simulink model "RLCCircuit"  (R2023b)
settings: Solver=VariableStepAuto  StartTime=0.0  StopTime=inf  MaxStep=1e-5  RelTol=1e-3
libraries: nesl_utility x6, fl_lib x4, ee_lib x3
settings Model: PacingRate=0.001000  Creator=Rocksmithed  LastModifiedBy=callie
settings DebuggingCC: UnconnectedInputMsg=warning  UnconnectedOutputMsg=warning  UnconnectedLineMsg=warning
settings ModelReferenceCC: EnableRefExpFcnMdlSchedulingChecks=on
settings RTWCC: DLArmComputeVersion=19.05

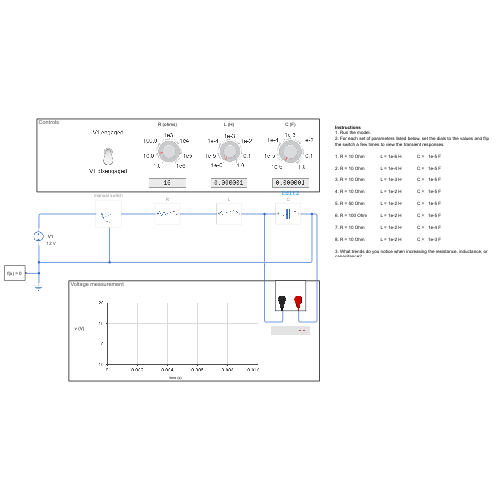
[thumbnail: Simulink's stored preview of the top-level diagram]
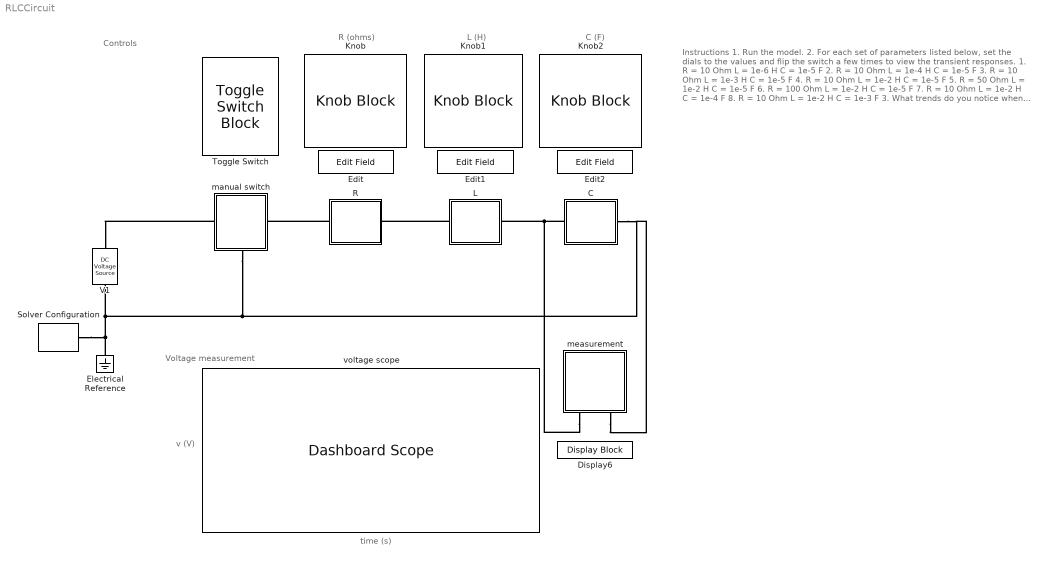
== system RLCCircuit ==
  note: R (ohms)
  note: Voltage measurement
  note: Instructions
      | 1. Run the model.
      | 2. For each set of parameters listed below, set the dials to the values and flip the switch a few times to view the transient responses.
      |
      | 1. R = 10 Ohm L = 1e-6 H C = 1e-5 F
      |
      | 2. R = 10 Ohm L = 1e-4 H C = 1e-5 F
      |
      | 3. R = 10 Ohm L = 1e-3 H C = 1e-5 F
      |
      | 4. R = 10 Ohm L = 1e-2 H C = 1e-5 F
      |
      | 5. R = 50 Ohm L = 1e-2 H C = 1e-5 F
      |
      | 6. R = 100 Ohm L = 1e-2 H C = 1e-5 F
      |
      | 7. R = 10 Ohm L = 1e-2 H C = 1e-4 F
      |
      | 8. R = 10 Ohm L = 1e-2 H C = 1e-3 F
      |
      | 3. What trends do you notice when increasing the resistance, inductance, or capacitance?
  note: time (s)
  note: v (V)
  note: Controls
  note: L (H)
  note: C (F)
  C : Subsystem
      mask Display: image('variablecapacitor.png');
  Display6 : DisplayBlock  LabelPosition=Hide  Format=Custom  Alignment=Right  Transparency=1  FormatString=%0.4f
  Edit : EditField  LabelPosition=Hide  ShowInitialText=on  Alignment=Center
  Edit1 : EditField  LabelPosition=Hide  ShowInitialText=on  Alignment=Center
  Edit2 : EditField  LabelPosition=Hide  ShowInitialText=on  Alignment=Center
  Electrical Reference : fl_lib/Electrical/Electrical Elements/Electrical Reference
  Knob : KnobBlock  LabelPosition=Hide  ScaleMin=1  ScaleMax=1e6  ScaleType=Log
  Knob1 : KnobBlock  LabelPosition=Hide  ScaleMin=1e-6  ScaleMax=1  ScaleType=Log
  Knob2 : KnobBlock  LabelPosition=Hide  ScaleMin=1e-6  ScaleMax=1  ScaleType=Log
  L : Subsystem
      mask Display: image('variableinductor.png');
  R : Subsystem
      mask Display: image('variableresistor.png');
  Solver Configuration : nesl_utility/Solver Configuration  PhysicalDomain=network_engine_domain  SubClassName=solver  LeftPortType=input  RightPortType=generic  Tones=[]  Harmonics=[]  SimulateNoise=off  Profile=off  UseLocalSampling=off  EnableSwitchedLinearOptims=on  FrequencyDomain=off  UseCCode=off  RelTol=0.001  AbsTol=1e-06  MinStep=1e-09  ToWorkspace=off  RevertToSquareIcSolve=off  NumHomotopyIterations=100  PhasorMode=off  PhasorModeNumHarmonics=1  ConsistencySolver=NEWTON_FTOL  IndexReductionMethod=DerivativeReplacement  DoDC=off  ResidualTolerance=1e-09  ConsistencyTolSource=GLOBAL  ConsistencyAbsTol=0.001  ConsistencyRelTol=0.001  ConsistencyTolFactor=0.001  UseLocalSolver=off  LocalSolverChoice=NE_BACKWARD_EULER_ADVANCER  ResolveIndetEquations=on  FunctionEvalNumThread=1  LocalSolverSampleTime=0.001  DoFixedCost=off  MaxNonlinIter=3  MaxModeIter=2  ComputeImpulses=off  ImpulseIterations=2  LinearAlgebra=auto  LinearAlgebraNumThread=0  EquationFormulation=NE_TIME_EF  DelaysMemoryBudget=1024  AutomaticFiltering=on  FilteringTimeConstant=0.001  PartitionStorageMethod=AS_NEEDED  PartitionMemoryBudget=1024  PartitionMethod=ROBUST  MultibodyUseLocalSolver=off  MultibodyLocalSolverChoice=ODE1  MultibodyLocalSolverSampleTime=0.001
  Toggle Switch : ToggleSwitchBlock  LabelPosition=Hide
      settings: Values={{'V1 disengaged', 'V1 engaged'}, [0 1]}
  V1 : fl_lib/Electrical/Electrical Sources/DC Voltage Source  v0=12 V
      settings: AttributesFormatString=%<v0> %<v0_unit>
  manual switch : Subsystem
      settings: PortSchema="{\"entries\":[{\"content\":{\"sides\":[{\"content\":{\"connectorIds\":[\"LConn1\"]},\"type\":\"ConnectorPlacement.EquallySpacedRectSide\",\"uuid\":\"0e8d165f-9423-448d-a092-8a5aaec0f3f9\"},{\"content\":{\"connectorIds\":[\"RConn1\"],\"side\":\"RIGHT\"},\"type\":\"ConnectorPlacement.EquallySpacedRectSide\",\"uuid\":\"3a6701ab-7127-4025-a8cd-0b0ce6beee28\"},{\"content\":{\"connectorIds\":[],\"side\":\"TOP\"},\"type\":\"ConnectorPlacement.EquallySpacedRectSide\",\"uuid\":\"c8b7dcbe-92e8-45dd-b18b-fd43e016b5cf\"},{\"content\":{\"connectorIds\":[\"RConn2\"],\"side\":\"BOTTOM\"},\"type\":\"ConnectorPlacement.EquallySpacedRectSide\",\"uuid\":\"e38a5957-407c-408e-8d09-8d531b6a67a5\"}]},\"type\":\"ConnectorPlacement.EquallySpacedConnector\",\"uuid\":\"663f5a3e-52b5-405d-b6e3-1aa4958c6787\"}],\"packageUris\":[\"http://schema.mathworks.com/mf0/Connector/R2020b\"],\"version\":\"1.0\"}"
      mask Display: image('$imagefile'); % Use "Edit Image" on toolstrip to change.
  measurement : Subsystem
      settings: PortSchema="{\"entries\":[{\"content\":{\"sides\":[{\"content\":{\"connectorIds\":[]},\"type\":\"ConnectorPlacement.EquallySpacedRectSide\",\"uuid\":\"e6ae0c61-2eb5-460e-b2a2-38a9147b4757\"},{\"content\":{\"connectorIds\":[],\"side\":\"RIGHT\"},\"type\":\"ConnectorPlacement.EquallySpacedRectSide\",\"uuid\":\"ce3a3055-ccd0-4b2b-b818-955585f278b2\"},{\"content\":{\"connectorIds\":[\"LConn1\",\"LConn2\"],\"side\":\"TOP\"},\"type\":\"ConnectorPlacement.EquallySpacedRectSide\",\"uuid\":\"55693832-da2d-47ee-8c0b-c43271958a5d\"},{\"content\":{\"connectorIds\":[],\"side\":\"BOTTOM\"},\"type\":\"ConnectorPlacement.EquallySpacedRectSide\",\"uuid\":\"6e1fba19-6c00-4aec-b19d-3a06ce7f1244\"}]},\"type\":\"ConnectorPlacement.EquallySpacedConnector\",\"uuid\":\"91498f30-f262-43a8-9075-3f461cadc22e\"}],\"packageUris\":[\"http://schema.mathworks.com/mf0/Connector/R2020b\"],\"version\":\"1.0\"}"
      mask Display: image('leads.png'); % Use "Edit Image" on toolstrip to change.
  voltage scope : DashboardScope  ShowInitialText=off  TimeSpan=0.01  Ymin=-10  Ymax=20  ScaleAtStop=off
  connections:
  manual switch/RConn1 -- V1/LConn1
  Electrical Reference/LConn1 -- Solver Configuration/RConn1 -- C/RConn1 -- measurement/LConn1 -- manual switch/RConn2 -- V1/RConn1
  C/LConn1 -- L/RConn1 -- measurement/LConn2
  R/LConn1 -- manual switch/LConn1
  L/LConn1 -- R/RConn1

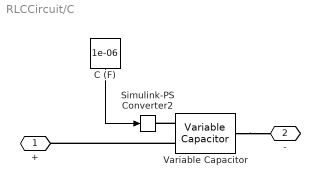
== system RLCCircuit/C ==
  C (F) : Constant  Value=1e-06
  Simulink-PS Converter2 : nesl_utility/Simulink-PS Converter  PhysicalDomain=network_engine_domain  SubClassName=ps_input  LeftPortType=input  RightPortType=output  PseudoPeriodic=off  Frequencies=[]  NoiseDistribution=none  NoiseParameters=[]  Unit=F  AffineConversion=off  FilteringAndDerivatives=provide  SimscapeFilterOrder=1  InputFilterTimeConstant=0.001  UdotUserProvided=0
  Variable Capacitor : ee_lib/Passive/Variable Capacitor  prm=2  Cmin=1e-9 F  r=1e-6 Ohm  v0=0 V  q0=0 C
      settings: InternalSimscapePortConfiguration="{\"Bottom\":[],\"Left\":[{\"id\":\"C\",\"label\":\"C\",\"type\":\"input\"},{\"id\":\"p\",\"label\":\"+\",\"type\":\"foundation.electrical.electrical\"}],\"Right\":[{\"id\":\"n\",\"label\":\"-\",\"type\":\"foundation.electrical.electrical\"}],\"Top\":[]}"
  + : PMIOPort  Side=Left
  - : PMIOPort  Port=2  Side=Right
  wires:
  C (F)/1 -> Simulink-PS Converter2/1
  connections:
  Variable Capacitor/LConn2 -- +/RConn1
  Variable Capacitor/LConn1 -- Simulink-PS Converter2/RConn1
  Variable Capacitor/RConn1 -- -/RConn1

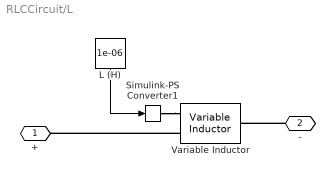
== system RLCCircuit/L ==
  L (H) : Constant  Value=1e-06
  Simulink-PS Converter1 : nesl_utility/Simulink-PS Converter  PhysicalDomain=network_engine_domain  SubClassName=ps_input  LeftPortType=input  RightPortType=output  PseudoPeriodic=off  Frequencies=[]  NoiseDistribution=none  NoiseParameters=[]  Unit=H  AffineConversion=off  FilteringAndDerivatives=provide  SimscapeFilterOrder=1  InputFilterTimeConstant=0.001  UdotUserProvided=0
  Variable Inductor : ee_lib/Passive/Variable Inductor  prm=1  Lmin=1e-6 H  g=1e-9 1/Ohm  i0=0 A  phi0=0 Wb
      settings: InternalSimscapePortConfiguration="{\"Bottom\":[],\"Left\":[{\"id\":\"L\",\"label\":\"L\",\"type\":\"input\"},{\"id\":\"p\",\"label\":\"+\",\"type\":\"foundation.electrical.electrical\"}],\"Right\":[{\"id\":\"n\",\"label\":\"-\",\"type\":\"foundation.electrical.electrical\"}],\"Top\":[]}"
  + : PMIOPort  Side=Left
  - : PMIOPort  Port=2  Side=Right
  wires:
  L (H)/1 -> Simulink-PS Converter1/1
  connections:
  Simulink-PS Converter1/RConn1 -- Variable Inductor/LConn1
  -/RConn1 -- Variable Inductor/RConn1
  Variable Inductor/LConn2 -- +/RConn1

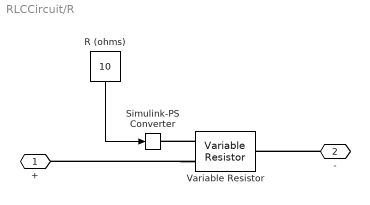
== system RLCCircuit/R ==
  " R (ohms)" : Constant  Value=10
  Simulink-PS Converter : nesl_utility/Simulink-PS Converter  PhysicalDomain=network_engine_domain  SubClassName=ps_input  LeftPortType=input  RightPortType=output  PseudoPeriodic=off  Frequencies=[]  NoiseDistribution=none  NoiseParameters=[]  Unit=Ohm  AffineConversion=off  FilteringAndDerivatives=provide  SimscapeFilterOrder=1  InputFilterTimeConstant=0.001  UdotUserProvided=0
  Variable Resistor : fl_lib/Electrical/Electrical Elements/Variable Resistor  Rmin=0 Ohm  thermalEnable=false  thermal_mass=1 J/K  i_specify=off  i_priority=None  i=0 A  i_nominal_specify=off  i_nominal_unit=A  i_nominal_value=1  v_specify=off  v_priority=None  v=0 V  v_nominal_specify=off  v_nominal_unit=V  v_nominal_value=1  T_specify=off  T_priority=None  T=300 K  T_nominal_specify=off  T_nominal_unit=K  T_nominal_value=1
  + : PMIOPort  Side=Left
  - : PMIOPort  Port=2  Side=Right
  wires:
  " R (ohms)"/1 -> Simulink-PS Converter/1
  connections:
  Variable Resistor/LConn1 -- Simulink-PS Converter/RConn1
  -/RConn1 -- Variable Resistor/RConn1
  Variable Resistor/LConn2 -- +/RConn1

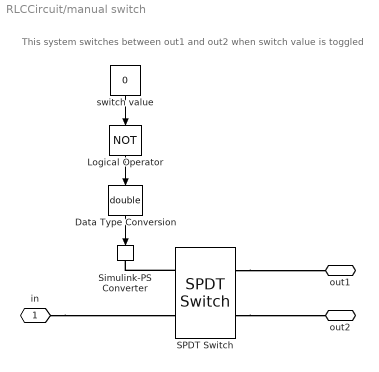
== system RLCCircuit/manual switch ==
  note: This system switches between out1 and out2 when switch value is toggled
  Data Type Conversion : DataTypeConversion  OutDataTypeStr=double  SaturateOnIntegerOverflow=off  RndMeth=Floor
  Logical Operator : Logic  Operator=NOT  AllPortsSameDT=off  OutDataTypeStr=boolean
  SPDT Switch : ee_lib/Switches & Breakers/SPDT Switch  R_closed=0.01 Ohm  G_open=1e-6 S  Threshold=0.5 V  Width=0 V  model_dynamics=0  t_on=1e-3 s  t_off=1e-3 s  initial_vT=0 V
  Simulink-PS Converter : nesl_utility/Simulink-PS Converter  PhysicalDomain=network_engine_domain  SubClassName=ps_input  LeftPortType=input  RightPortType=output  PseudoPeriodic=off  Frequencies=[]  NoiseDistribution=none  NoiseParameters=[]  Unit=1  AffineConversion=off  FilteringAndDerivatives=provide  SimscapeFilterOrder=1  InputFilterTimeConstant=0.001  UdotUserProvided=0
  switch value : Constant  Value=0
  in : PMIOPort  Side=Left
  out1 : PMIOPort  Port=2  Side=Right
  out2 : PMIOPort  Port=3  Side=Right
  wires:
  Data Type Conversion/1 -> Simulink-PS Converter/1
  Logical Operator/1 -> Data Type Conversion/1
  switch value/1 -> Logical Operator/1
  connections:
  SPDT Switch/LConn1 -- Simulink-PS Converter/RConn1
  in/RConn1 -- SPDT Switch/LConn2
  SPDT Switch/RConn1 -- out1/RConn1
  SPDT Switch/RConn2 -- out2/RConn1

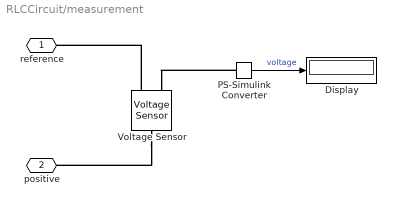
== system RLCCircuit/measurement ==
  Display : Display
  PS-Simulink Converter : nesl_utility/PS-Simulink Converter  PhysicalDomain=network_engine_domain  SubClassName=ps_output  LeftPortType=input  RightPortType=output  PseudoPeriodic=off  Frequencies=[]  VectorFormat=1-D array  Unit=V  AffineConversion=off
  Voltage Sensor : fl_lib/Electrical/Electrical Sensors/Voltage Sensor
  reference : PMIOPort  Side=Left
  positive : PMIOPort  Port=2  Side=Left
  wires:
  PS-Simulink Converter/1 -> Display/1  "voltage"
  connections:
  PS-Simulink Converter/LConn1 -- Voltage Sensor/RConn1
  Voltage Sensor/LConn1 -- positive/RConn1
  Voltage Sensor/RConn2 -- reference/RConn1
